simulink model "Week2_Sum3"  (R2020b)
settings: Solver=VariableStepAuto  StartTime=0.0  StopTime=5  RelTol=1e-3
settings Model: Creator=Aradhana desai  LastModifiedBy=Aradhana desai

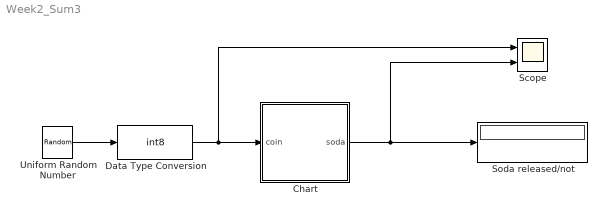
== system Week2_Sum3 ==
  Chart : Stateflow chart  TreatAsAtomicUnit=on
  Data Type Conversion : DataTypeConversion  OutDataTypeStr=int8  RndMeth=Nearest  SaturateOnIntegerOverflow=on
  Scope : Scope  NumInputPorts=2
  Soda released/not : Display
  Uniform Random Number : UniformRandomNumber  Minimum=0  Maximum=2  Seed=337  SampleTime=10
  wires:
  Chart/1(soda) -> Scope/2, Soda released/not/1
  Data Type Conversion/1 -> Scope/1, Chart/1(coin)
  Uniform Random Number/1 -> Data Type Conversion/1

== stateflow chart Week2_Sum3/Chart ==
  state got_0
  state got_nickel
  state got_dime
  (default) -> got_0
  got_0 -> got_nickel [order 1] : [coin==1]{soda=0}
  got_nickel -> got_0 [order 2] : [coin==2]{soda=1}
  got_dime -> got_0 [order 1] : [coin==1]{soda=1}
  got_0 -> got_dime [order 2] : [coin==2]{soda=0}
  got_dime -> got_nickel [order 2] : [coin==2]{soda=1}
  got_nickel -> got_dime [order 1] : [coin==1]{soda=0}
  data: soda output; coin input
